simulink model "pv_battery_converter_simulation"  (R2012b)
settings: Solver=ode45  StartTime=0.0  StopTime=3600*14  FixedStep=0.01  RelTol=1e-3
values from neighbouring files (symbols this model uses):
  b = [b1 b2]    [battery_model.m]
  c = p    [converter_model.m]
  G_to_PpvMax = [G_to_PpvMax; G_vec(i) Ppv_use(end)]    [make_pv_characteristics_table.m]
  G_vec = [min(G_log(:,2)):(max(G_log(:,2)) - min(G_log(:,2)))/49:max(G_log(:,2))]/1000    [make_pv_characteristics_table.m]
  H = 10    [make_pv_characteristics_table.m]
  Ppv_to_Ipv = []    [make_pv_characteristics_table.m]
  Ppv_vec = [Ppv_min: (Ppv_max - Ppv_min)/200: Ppv_max]    [make_pv_characteristics_table.m]
  startSOC = 0.5    [battery_model.m]
  W = 1    [make_pv_characteristics_table.m]
libraries: simulink x2
settings Model: Creator=dhshin  LastModifiedBy=simo
settings DataIOCC: ExternalInput=[c,b]  SignalLoggingSaveFormat=ModelDataLogs
settings DebuggingCC: FcnCallInpInsideContextMsg=EnableAllAsWarning
settings GRTTargetCC: CombineOutputUpdateFcns=off  GRTInterface=on
settings ConfigurationSet: Description=SimMechanics 2G

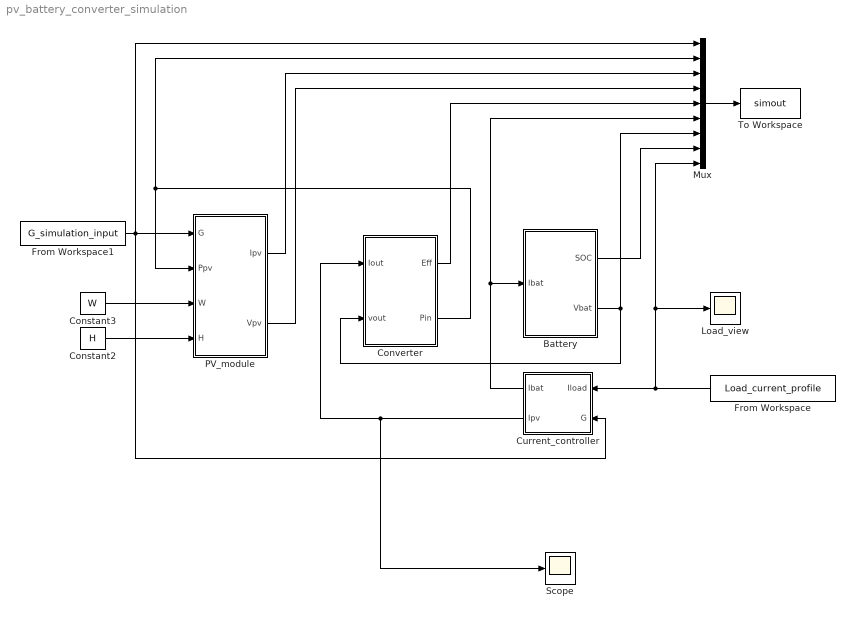
== system pv_battery_converter_simulation ==
  Battery : Subsystem
  Constant2 : Constant  Value=H
  Constant3 : Constant  Value=W
  Converter : Subsystem
  Current_controller : Subsystem
  From Workspace : FromWorkspace  VariableName=Load_current_profile  SampleTime=0
  From Workspace1 : FromWorkspace  VariableName=G_simulation_input  SampleTime=0
  Load_view : Scope
      settings: TimeRange=100000  YMin=12.5  YMax=17  SaveName=ScopeData6
  Mux : Mux  Inputs=9
  PV_module : Subsystem
  Scope : Scope
      settings: TimeRange=2878.93864013267  YMin=0.3142969984202212  YMax=0.318088467614534  SaveName=ipv_req
  To Workspace : ToWorkspace  VariableName=simout  SampleTime=-1  SaveFormat=Structure With Time
  wires:
  From Workspace1/1 -> PV_module/1(G), Mux/1, Current_controller/2(G)
  Mux/1 -> To Workspace/1
  Constant2/1 -> PV_module/4(H)
  Constant3/1 -> PV_module/3(W)
  From Workspace/1 -> Mux/9, Load_view/1, Current_controller/1(Iload)
  Current_controller/1(Ibat) -> Battery/1(Ibat), Mux/6
  Current_controller/2(Ipv) -> Scope/1, Converter/1(Iout)
  Battery/2(Vbat) -> Mux/7, Converter/2(vout)
  PV_module/2(Vpv) -> Mux/4
  Converter/2(Pin) -> PV_module/2(Ppv), Mux/2
  PV_module/1(Ipv) -> Mux/3
  Converter/1(Eff) -> Mux/5
  Battery/1(SOC) -> Mux/8

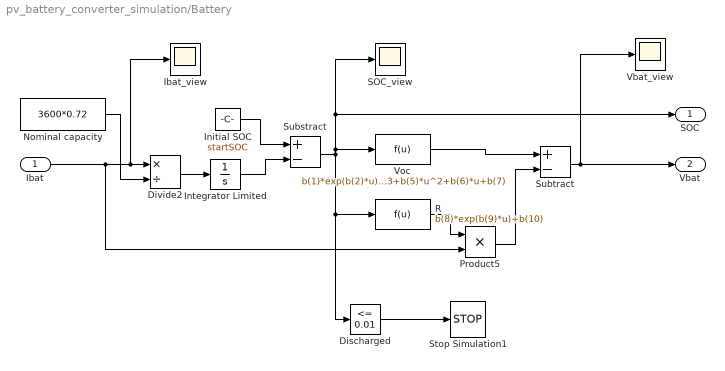
== system pv_battery_converter_simulation/Battery ==
  Ibat : Inport
  Discharged : simulink/Logic and Bit Operations/Compare To Constant  relop=<=  const=0.01  OutDataTypeStr=boolean  ZeroCross=off
  Divide2 : Product  Inputs=*/
  Ibat_view : Scope
      settings: TimeRange=100000  YMin=12.5  YMax=17  SaveName=Ibat_view
  Initial SOC : Constant  Value=startSOC
  Integrator Limited : Integrator  LimitOutput=on  UpperSaturationLimit=startSOC  LowerSaturationLimit=-1+startSOC
  Nominal capacity : Constant  Value=3600*0.72
  Product5 : Product  RndMeth=Zero
  R : Fcn  Expr=b(8)*exp(b(9)*u)+b(10)
  SOC_view : Scope
      settings: SaveName=SOC_view
  Stop Simulation1 : Stop
  Substract : Sum  Inputs=+-
  Subtract : Sum  Inputs=+-
  Vbat_view : Scope
      settings: TimeRange=100000  YMin=12.5  YMax=17  SaveName=Vbat_view
  Voc : Fcn  Expr=b(1)*exp(b(2)*u)+b(3)*u^4+b(4)*u^3+b(5)*u^2+b(6)*u+b(7)
  SOC : Outport
  Vbat : Outport  Port=2
  wires:
  Ibat/1 -> Product5/2, Divide2/1, Ibat_view/1
  Substract/1 -> Voc/1, SOC_view/1, SOC/1, R/1, Discharged/1
  Product5/1 -> Subtract/2
  Subtract/1 -> Vbat/1, Vbat_view/1
  R/1 -> Product5/1
  Voc/1 -> Subtract/1
  Nominal capacity/1 -> Divide2/2
  Divide2/1 -> Integrator Limited/1
  Integrator Limited/1 -> Substract/2
  Initial SOC/1 -> Substract/1
  Discharged/1 -> Stop Simulation1/1

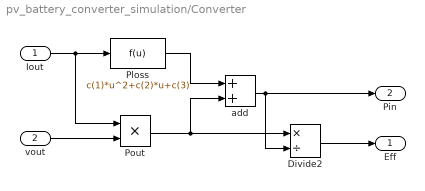
== system pv_battery_converter_simulation/Converter ==
  Iout : Inport
  vout : Inport  Port=2
  Divide2 : Product  Inputs=*/
  Ploss : Fcn  Expr=c(1)*u^2+c(2)*u+c(3)
  Pout : Product  RndMeth=Zero
  add : Sum
  Eff : Outport
  Pin : Outport  Port=2
  wires:
  Iout/1 -> Ploss/1, Pout/1
  vout/1 -> Pout/2
  Ploss/1 -> add/1
  Pout/1 -> add/2, Divide2/1
  add/1 -> Divide2/2, Pin/1
  Divide2/1 -> Eff/1

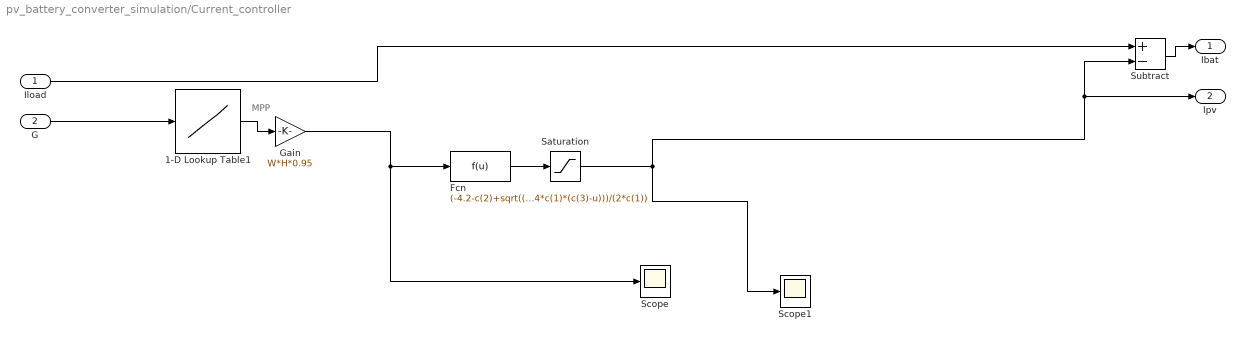
== system pv_battery_converter_simulation/Current_controller ==
  note: MPP
  Iload : Inport
  G : Inport  Port=2
  1-D Lookup Table1 : Lookup_n-D  NumberOfTableDimensions=1  BreakpointsForDimension1=G_to_PpvMax(:,1)  Table=G_to_PpvMax(:,2)  RndMeth=Simplest  InputSameDT=on
  Fcn : Fcn  Expr=(-4.2-c(2)+sqrt((4.2+c(2))^2-4*c(1)*(c(3)-u)))/(2*c(1))
  Gain : Gain  Gain=W*H*0.95
  Saturation : Saturate  UpperLimit=inf  LowerLimit=0
  Scope : Scope
  Scope1 : Scope
      settings: SaveName=ScopeData2
  Subtract : Sum  Inputs=+-
  Ibat : Outport
  Ipv : Outport  Port=2
  wires:
  G/1 -> 1-D Lookup Table1/1
  Iload/1 -> Subtract/1
  Subtract/1 -> Ibat/1
  Saturation/1 -> Scope1/1, Subtract/2, Ipv/1
  1-D Lookup Table1/1 -> Gain/1
  Fcn/1 -> Saturation/1
  Gain/1 -> Fcn/1, Scope/1

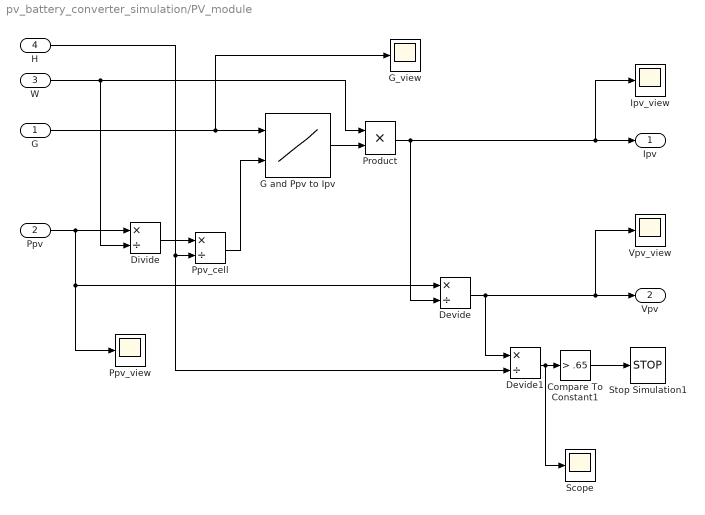
== system pv_battery_converter_simulation/PV_module ==
  G : Inport
  Ppv : Inport  Port=2
  W : Inport  Port=3
  H : Inport  Port=4
  Compare To Constant1 : simulink/Logic and Bit Operations/Compare To Constant  relop=>  const=.65  OutDataTypeStr=boolean  ZeroCross=off
  Devide : Product  Inputs=*/
  Devide1 : Product  Inputs=*/
  Divide : Product  Inputs=*/
  G and Ppv to Ipv : Lookup_n-D  BreakpointsForDimension1=G_vec  BreakpointsForDimension2=Ppv_vec  Table=Ppv_to_Ipv(:,:,3)  RndMeth=Simplest  InputSameDT=on
  G_view : Scope
      settings: TimeRange=52200  YMin=0.955  YMax=1.02
  Ipv_view : Scope
      settings: TimeRange=100000  YMin=-2  YMax=12  SaveName=Ipv_view
  Ppv_cell : Product  Inputs=*/
  Ppv_view : Scope
      settings: TimeRange=100000  YMin=-2  YMax=12  SaveName=ScopeData5
  Product : Product  RndMeth=Zero
  Scope : Scope
      settings: SaveName=ScopeData3
  Stop Simulation1 : Stop
  Vpv_view : Scope
      settings: TimeRange=100000  YMin=7  YMax=12  SaveName=Vpv_view
  Ipv : Outport
  Vpv : Outport  Port=2
  wires:
  Compare To Constant1/1 -> Stop Simulation1/1
  G/1 -> G and Ppv to Ipv/1, G_view/1
  G and Ppv to Ipv/1 -> Product/2
  Product/1 -> Devide/2, Ipv/1, Ipv_view/1
  Ppv/1 -> Divide/1, Devide/1, Ppv_view/1
  Ppv_cell/1 -> G and Ppv to Ipv/2
  Divide/1 -> Ppv_cell/1
  W/1 -> Divide/2, Product/1
  H/1 -> Ppv_cell/2, Devide1/2
  Devide/1 -> Vpv/1, Vpv_view/1, Devide1/1
  Devide1/1 -> Scope/1, Compare To Constant1/1
